simulink subsystem "Actuator"  (R2022b)
settings: Solver=VariableStepAuto  StartTime=0.0  StopTime=10.0  RelTol=1e-3
undefined symbols (not defined in the file): J_gearbox_1, J_gearbox_2, L, R
settings Model: Creator=Maxim Kozlov  LastModifiedBy=KozlovM
settings OptimizationCC: ReuseModelBlockBuffer=on

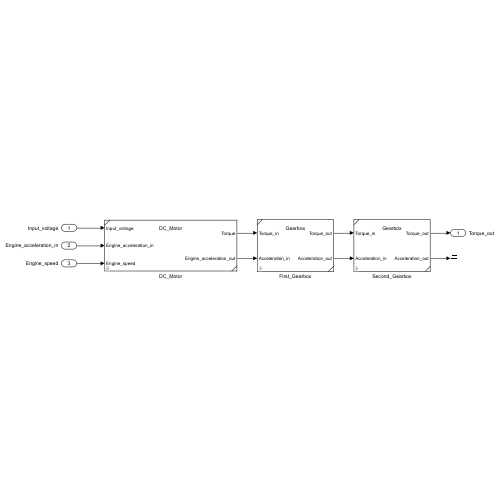
[thumbnail: Simulink's stored preview of the top-level diagram]
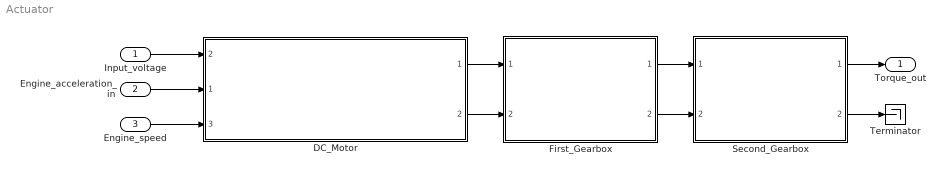
== system Actuator ==
  Input_voltage : Inport
  Engine_acceleration_in : Inport  Port=2
  Engine_speed : Inport  Port=3
  DC_Motor : Subsystem  ReferencedSubsystem=DC_Motor  Km=Km  Kw=Kw  R=R  L=L  J_engine=J_engine
      settings: PortSchema="{\"entries\":[{\"content\":{\"sides\":[{\"content\":{\"connectorIds\":[\"In2\",\"In1\",\"In3\"]},\"type\":\"ConnectorPlacement.EquallySpacedRectSide\",\"uuid\":\"95acf8b1-32ed-469b-a5a0-31a29a62b015\"},{\"content\":{\"connectorIds\":[\"Out1\",\"Out2\"],\"side\":\"RIGHT\"},\"type\":\"ConnectorPlacement.EquallySpacedRectSide\",\"uuid\":\"424bca10-54c8-45c3-b4a3-7b161530ad58\"},{\"content\":{\"connectorIds\":[],\"side\":\"TOP\"},\"type\":\"ConnectorPlacement.EquallySpacedRectSide\",\"uuid\":\"38be544a-552a-435f-925c-7f69ffd89de6\"}]},\"type\":\"ConnectorPlacement.EquallySpacedConnector\",\"uuid\":\"f80823b3-c4e0-44f6-8ba8-2679ad72186a\"}],\"packageUris\":[\"http://schema.mathworks.com/mf0/Connector/R2020b\"],\"version\":\"1.0\"}"
  First_Gearbox : Subsystem  ReferencedSubsystem=Gearbox  i=i_gearbox_1  J=J_gearbox_1
  Second_Gearbox : Subsystem  ReferencedSubsystem=Gearbox  i=i_gearbox_2  J=J_gearbox_2
  Terminator : Terminator
  Torque_out : Outport
  wires:
  Engine_acceleration_in/1 -> DC_Motor/1
  Engine_speed/1 -> DC_Motor/3
  DC_Motor/1 -> First_Gearbox/1
  Input_voltage/1 -> DC_Motor/2
  DC_Motor/2 -> First_Gearbox/2
  First_Gearbox/1 -> Second_Gearbox/1
  First_Gearbox/2 -> Second_Gearbox/2
  Second_Gearbox/1 -> Torque_out/1
  Second_Gearbox/2 -> Terminator/1
